simulink model "topoint_pp"  (R2020a)
settings: Solver=FixedStepAuto  StartTime=0.0  StopTime=20  FixedStep=.01  RelTol=1e-3
undefined symbols (not defined in the file or in its folder): angdiff
libraries: simulink x2
settings Model: Creator=Jamie  LastModifiedBy=Jamie

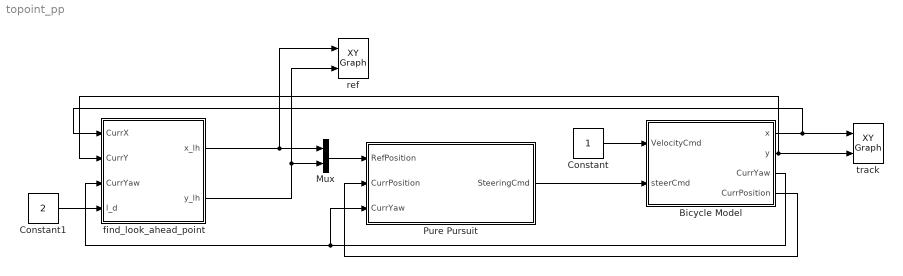
== system topoint_pp ==
  Bicycle Model : Subsystem
  Constant : Constant
  Constant1 : Constant  Value=2
  Mux : Mux  Inputs=2
  Pure Pursuit : Subsystem
  find_look_ahead_point : MATLAB Function  TreatAsAtomicUnit=on
  ref : simulink/Sinks/XY Graph  xmin=-1  xmax=15  ymin=-1  ymax=10  st=-1
  track : simulink/Sinks/XY Graph  xmin=0  xmax=10  ymin=0  ymax=10  st=-1
  wires:
  Mux/1 -> Pure Pursuit/1(RefPosition)
  Bicycle Model/4(CurrPosition) -> Pure Pursuit/2(CurrPosition)
  Pure Pursuit/1(SteeringCmd) -> Bicycle Model/2(steerCmd)
  Bicycle Model/3(CurrYaw) -> Pure Pursuit/3(CurrYaw), find_look_ahead_point/3(CurrYaw)
  Bicycle Model/1(x) -> find_look_ahead_point/1(CurrX), track/1
  Bicycle Model/2(y) -> find_look_ahead_point/2(CurrY), track/2
  Constant/1 -> Bicycle Model/1(VelocityCmd)
  find_look_ahead_point/1(x_lh) -> ref/1, Mux/1
  find_look_ahead_point/2(y_lh) -> ref/2, Mux/2
  Constant1/1 -> find_look_ahead_point/4(l_d)

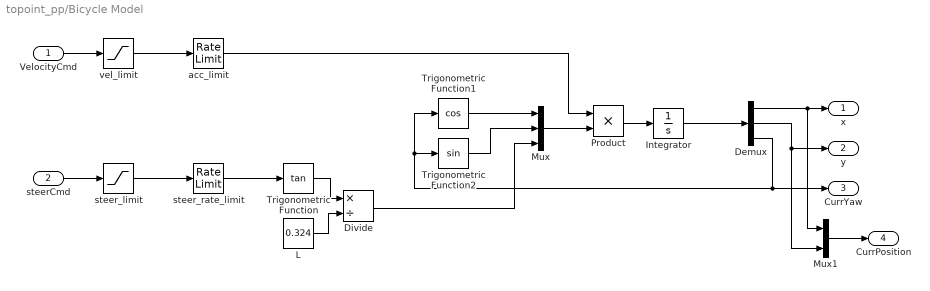
== system topoint_pp/Bicycle Model ==
  VelocityCmd : Inport
  steerCmd : Inport  Port=2
  Demux : Demux  Outputs=3
  Divide : Product  Inputs=*/
  Integrator : Integrator  InitialCondition=[1, 0, pi/2]
  L : Constant  Value=0.324
  Mux : Mux  Inputs=3
  Mux1 : Mux  Inputs=2
  Product : Product
  Trigonometric Function : Trigonometry  Operator=tan
  Trigonometric Function1 : Trigonometry  Operator=cos
  Trigonometric Function2 : Trigonometry
  acc_limit : RateLimiter  SampleTimeMode=inherited
  steer_limit : Saturate
  steer_rate_limit : RateLimiter  RisingSlewLimit=3  FallingSlewLimit=-3  SampleTimeMode=inherited
  vel_limit : Saturate  UpperLimit=3  LowerLimit=-3
  x : Outport
  y : Outport  Port=2
  CurrYaw : Outport  Port=3
  CurrPosition : Outport  Port=4
  wires:
  steerCmd/1 -> steer_limit/1
  VelocityCmd/1 -> vel_limit/1
  vel_limit/1 -> acc_limit/1
  steer_limit/1 -> steer_rate_limit/1
  steer_rate_limit/1 -> Trigonometric Function/1
  Trigonometric Function/1 -> Divide/1
  L/1 -> Divide/2
  acc_limit/1 -> Product/1
  Trigonometric Function1/1 -> Mux/1
  Trigonometric Function2/1 -> Mux/2
  Mux/1 -> Product/2
  Product/1 -> Integrator/1
  Divide/1 -> Mux/3
  Integrator/1 -> Demux/1
  Demux/1 -> Mux1/1, x/1
  Demux/2 -> Mux1/2, y/1
  Demux/3 -> Trigonometric Function1/1, Trigonometric Function2/1, CurrYaw/1
  Mux1/1 -> CurrPosition/1

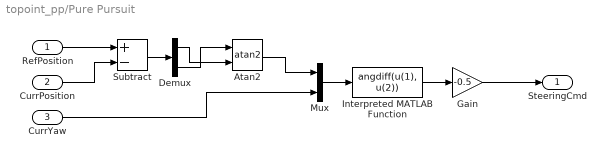
== system topoint_pp/Pure Pursuit ==
  RefPosition : Inport
  CurrPosition : Inport  Port=2
  CurrYaw : Inport  Port=3
  Atan2 : Trigonometry  Operator=atan2
  Demux : Demux  Outputs=2
  Gain : Gain  Gain=-0.5
  Interpreted MATLAB Function : MATLABFcn  MATLABFcn=angdiff(u(1), u(2))
  Mux : Mux  Inputs=2
  Subtract : Sum  Inputs=+-
  SteeringCmd : Outport
  wires:
  RefPosition/1 -> Subtract/1
  CurrPosition/1 -> Subtract/2
  Subtract/1 -> Demux/1
  Demux/2 -> Atan2/1
  Demux/1 -> Atan2/2
  Mux/1 -> Interpreted MATLAB Function/1
  Atan2/1 -> Mux/1
  CurrYaw/1 -> Mux/2
  Interpreted MATLAB Function/1 -> Gain/1
  Gain/1 -> SteeringCmd/1

== matlab function topoint_pp/find_look_ahead_point ==
  data: CurrX input; x_lh output; y_lh output; CurrY input; CurrYaw input; l_d input
function [x_lh, y_lh] = fcn(CurrX,CurrY,CurrYaw,l_d)
x = (0:0.01:15);
% y = -0.1*x.*x + 2*x;
y = 10*sin(pi/10*x);

% CurrX = 1;
% CurrY = 1;
% CurrYaw = 0;
% l_d = 1;
% 
x_r = x;
y_r = y;

for i = 1:1501
    x_r(i) = (x(i) - CurrX)*cos(CurrYaw) + (y(i) - CurrY)*sin(CurrYaw);
    y_r(i) = (y(i) - CurrY)*cos(CurrYaw) - (x(i) - CurrX)*sin(CurrYaw);
end

j = 1;
while(x_r(j)<0)
    j = j + 1;
    if j == 1501
        break
    end
end
k = j;

% while(sqrt(x_r(k)*x_r(k) + y_r(k)*y_r(k)) < l_d)
%     if k < 1001
%         k = k + 1;
%     else
%         k = 1001;
%         break
%     end
% end
%     x_lh_r = x_r(k);
%     y_lh_r = y_r(k);

if(sqrt(x_r(k)*x_r(k) + y_r(k)*y_r(k)) < l_d)
    if(k <= 1501)
        while(1)
            k = k + 1;
            if(sqrt(x_r(k)*x_r(k) + y_r(k)*y_r(k)) > l_d)
                x_lh_r = x_r(k);
                y_lh_r = y_r(k);
                break
            end
            if(k > 1501)
                x_lh_r = 2;
                y_lh_r = 0;
                break
            end
        end
    else
        x_lh_r = 2;
        y_lh_r = 0;
    end
else
    x_lh_r = 2;
    y_lh_r = 0;
end
        
x_lh = x_lh_r*cos(-CurrYaw) + y_lh_r*sin(-CurrYaw) + CurrX;
y_lh = y_lh_r*cos(-CurrYaw) - x_lh_r*sin(-CurrYaw) + CurrY;
